simulink model "internal_PortLayout"  (R2016b)
settings: Solver=VariableStepAuto  StartTime=0.0  StopTime=10.0  RelTol=1e-3
settings Model: BOSCHToolsVersion=6.2  Creator=tkr5kor  LastModifiedBy=tkr5kor
settings SFSimCC: ModelFunctionsGlobalVisibility=off

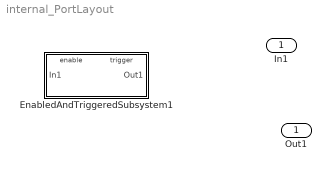
== system internal_PortLayout ==
  In1 : Inport
  EnabledAndTriggeredSubsystem1 : Subsystem  TreatAsAtomicUnit=on
      settings: RTWSystemCode=Inline
  Out1 : Outport

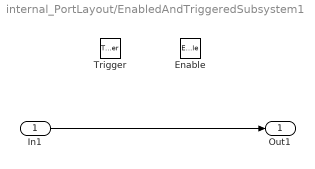
== system internal_PortLayout/EnabledAndTriggeredSubsystem1 ==
  In1 : Inport
  Enable : EnablePort
      settings: AttributesFormatString=%<StatesWhenEnabling>
  Trigger : TriggerPort  VariantControl=Variant
  Out1 : Outport
  wires:
  In1/1 -> Out1/1
